simulink model "Matlab_Function_1"  (R2021a)
settings: Solver=FixedStepDiscrete  StartTime=0.0  StopTime=inf  FixedStep=1e-3  RelTol=1e-3  EnableMultiTasking=on
libraries: arduinolib x8, simulink x1
settings Model: SILPILModeSetting=veronly  ExtModeTrigDuration=2  Creator=Admin  LastModifiedBy=Admin
settings OptimizationCC: EnhancedBackFolding=on  PassReuseOutputArgsAs=Individual arguments  ZeroExternalMemoryAtStartup=off  ZeroInternalMemoryAtStartup=off  MaxStackSize=64  OptimizeBlockOrder=speed  DifferentSizesBufferReuse=on  OptimizationCustomize=off  EfficientTunableParamExpr=on
settings DebuggingCC: ParameterTunabilityLossMsg=error
settings HardwareCC: ProdBitPerInt=16  ProdBitPerPointer=16  ProdBitPerSizeT=16  ProdBitPerPtrDiffT=16  ProdLargestAtomicFloat=None  ProdWordSize=8  ProdHWDeviceType=Atmel->AVR
settings SFSimCC: MATLABDynamicMemAlloc=off
settings RTWCC: SystemTargetFile=ert.tlc  HardwareBoard=Arduino Uno  TemplateMakefile=ert_default_tmf  Toolchain=Arduino AVR  BuildConfiguration=Faster Runs
settings CodeAppCC: ForceParamTrailComments=on  IgnoreCustomStorageClasses=off  OperatorAnnotations=on  SimulinkDataObjDesc=on  SFDataObjDesc=on  InsertBlockDesc=on
settings ERTTargetCC: SupportContinuousTime=on  SupportVariableSizeSignals=on  ExtModeStaticAllocSize=250

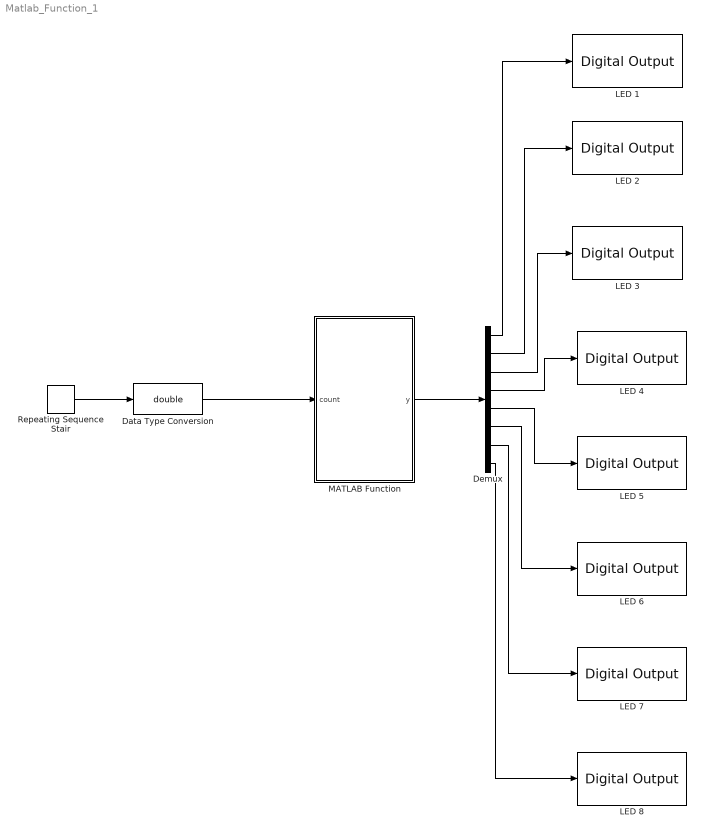
== system Matlab_Function_1 ==
  Data Type Conversion : DataTypeConversion  OutDataTypeStr=double
  Demux : Demux  Outputs=8
  LED 1 : arduinolib/Digital Output  pinNumber=10  Direction=output  blockPlatform=arduino
  LED 2 : arduinolib/Digital Output  pinNumber=9  Direction=output  blockPlatform=arduino
  LED 3 : arduinolib/Digital Output  pinNumber=8  Direction=output  blockPlatform=arduino
  LED 4 : arduinolib/Digital Output  pinNumber=7  Direction=output  blockPlatform=arduino
  LED 5 : arduinolib/Digital Output  pinNumber=6  Direction=output  blockPlatform=arduino
  LED 6 : arduinolib/Digital Output  pinNumber=5  Direction=output  blockPlatform=arduino
  LED 7 : arduinolib/Digital Output  pinNumber=4  Direction=output  blockPlatform=arduino
  LED 8 : arduinolib/Digital Output  pinNumber=3  Direction=output  blockPlatform=arduino
  MATLAB Function : MATLAB Function  TreatAsAtomicUnit=on
  Repeating Sequence Stair : simulink/Sources/Repeating Sequence Stair  OutValues=[0 1 2 3 4 5 6 7]  tsamp=0.5  OutMin=[]  OutMax=[]  OutDataTypeStr=double  OutputDataTypeScalingMode=double  OutDataType=fixdt(0,8)  ConRadixGroup=Best Precision: Vector-wise  OutScaling=2^-12
  wires:
  MATLAB Function/1(y) -> Demux/1
  Demux/1 -> LED 1/1
  Demux/2 -> LED 2/1
  Demux/3 -> LED 3/1
  Demux/4 -> LED 4/1
  Demux/5 -> LED 5/1
  Demux/6 -> LED 6/1
  Demux/7 -> LED 7/1
  Demux/8 -> LED 8/1
  Data Type Conversion/1 -> MATLAB Function/1(count)
  Repeating Sequence Stair/1 -> Data Type Conversion/1

== matlab function Matlab_Function_1/MATLAB Function ==
  data: count input; y output size=[1,8]
function y = LED_out(count)
y = [false, false, false, false, false, false, false, false];
y(count) = true;
